simulink model "three_phase_bridge_inversion"  (Simulink 6.1)
settings: Solver=ode23tb  StartTime=0.0  StopTime=0.1499  MaxStep=1e-4  RelTol=1e-3  AbsTol=.01
libraries: powerlib x12, powerlib_extras x1
settings Model: LastModifiedBy=ThinkPad
settings DebuggingCC: SolverPrmCheckMsg=warning

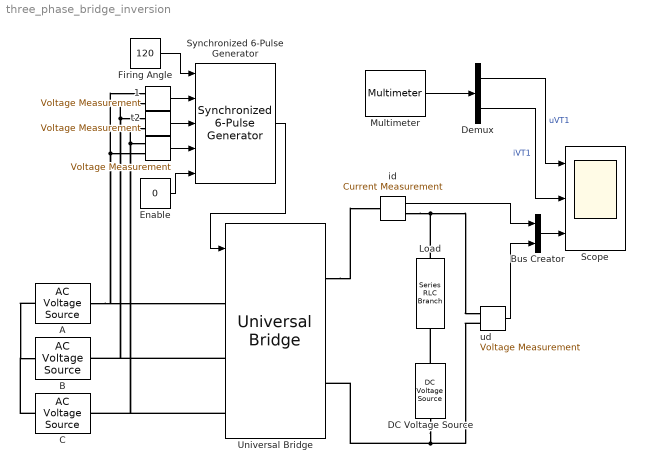
== system three_phase_bridge_inversion ==
  "   " : powerlib/Measurements/Voltage Measurement  PhasorSimulation=off  OutputType=Complex  PSBequivalent=0
  1 : powerlib/Measurements/Voltage Measurement  PhasorSimulation=off  OutputType=Complex  PSBequivalent=0
  A : powerlib/Electrical Sources/AC Voltage Source  Amplitude=100  Phase=30  Frequency=50  SampleTime=0  Measurements=None
  B : powerlib/Electrical Sources/AC Voltage Source  Amplitude=100  Phase=-90  Frequency=50  SampleTime=0  Measurements=None
  Bus Creator : BusCreator  DialogController=Simulink.DDGSource_Bus  Inputs=2
  C : powerlib/Electrical Sources/AC Voltage Source  Amplitude=100  Phase=-210  Frequency=50  SampleTime=0  Measurements=None
  DC Voltage Source : powerlib/Electrical Sources/DC Voltage Source  Orientation=down  Amplitude=200  Measurements=None
  Demux : Demux  Outputs=2
  Enable : Constant  Value=0
  Firing Angle : Constant  Value=120
  Load : powerlib/Elements/Series RLC Branch  Orientation=down  PhysicalDomain=powersysdomain  SubClassName=unknown  LeftPortType=p1  RightPortType=p1  LConnTagsString=__new0  RConnTagsString=__new0  Resistance=2  Inductance=0.01  Capacitance=inf  Measurements=None
  Multimeter : powerlib/Measurements/Multimeter  Tag=PoWeRsYsTeMmEaSuReMeNt  PhasorSimulation=off  OutputType=Magnitude  sel=[1 11]  L=16  Gain=[1 1]  yselected={'Usw1: Universal Bridge','Isw1: Universal Bridge'};  PSBOutputType=1  PSBequivalent=0  AxesSetting=[0,0.1,-100,100]  Display=0  SavedBlockNames=-11
      settings: AttributesFormatString=\n
  Scope : Scope  NumInputPorts=3
      settings: TimeRange=0.05  YMin=-200~0~-200  YMax=200~100~200  Decimation=5  SampleInput=on  SampleTime=1e-4
  Synchronized 6-Pulse Generator : powerlib_extras/Control  Blocks/Synchronized 6-Pulse Generator  freq=50  pwidth=10  Double_Pulse=on
  Universal Bridge : powerlib/Power Electronics/Universal Bridge  Arms=3  SnubberResistance=1e5  SnubberCapacitance=inf  Device=Thyristors  Ron=1e-3  Lon=0  ForwardVoltages="[  0  0  ]"  ForwardVoltage=0  GTOparameters=[ 10e-6 , 20e-6 ]  IGBTparameters=[ 1e-6 , 2e-6 ]  Measurements=All voltages and currents
  id : powerlib/Measurements/Current Measurement  PhasorSimulation=off  OutputType=Complex  PSBequivalent=0
  t2 : powerlib/Measurements/Voltage Measurement  PhasorSimulation=off  OutputType=Complex  PSBequivalent=0
  ud : powerlib/Measurements/Voltage Measurement  PhasorSimulation=off  OutputType=Complex  PSBequivalent=0
  wires:
  ud/1 -> Bus Creator/2
  1/1 -> Synchronized 6-Pulse Generator/2
  t2/1 -> Synchronized 6-Pulse Generator/3
  "   "/1 -> Synchronized 6-Pulse Generator/4
  Synchronized 6-Pulse Generator/1 -> Universal Bridge/1
  Firing Angle/1 -> Synchronized 6-Pulse Generator/1
  Enable/1 -> Synchronized 6-Pulse Generator/5
  id/1 -> Bus Creator/1
  Bus Creator/1 -> Scope/3
  Multimeter/1 -> Demux/1
  Demux/1 -> Scope/1  "uVT1"
  Demux/2 -> Scope/2  "iVT1"
  connections:
  id/RConn1 -- Load/LConn1 -- ud/LConn1
  A/LConn1 -- C/LConn1 -- B/LConn1
  Universal Bridge/LConn3 -- C/RConn1 -- t2/LConn2 -- "   "/LConn1
  Universal Bridge/LConn2 -- B/RConn1 -- 1/LConn2 -- t2/LConn1
  ud/LConn2 -- Universal Bridge/RConn2 -- DC Voltage Source/RConn1
  A/RConn1 -- Universal Bridge/LConn1 -- 1/LConn1 -- "   "/LConn2
  Universal Bridge/RConn1 -- id/LConn1
  DC Voltage Source/LConn1 -- Load/RConn1
